simulink model "Linearized_system_simulink"  (R2023b)
settings: Solver=VariableStepAuto  StartTime=0.0  StopTime=100  RelTol=1e-3
values from neighbouring files (symbols this model uses):
  K = place(A,B,[-1, -2, -3, -4])    [Linearized_system.m]
  theta0 = 60000/(m*g)    (= 0.0784129224496)    [Linearized_system.m]
  v0 = 840/3.6    (= 233.333333333)    [Linearized_system.m]
  w0 = 0    [Linearized_system.m]
settings Model: Creator=nasir  LastModifiedBy=nasir

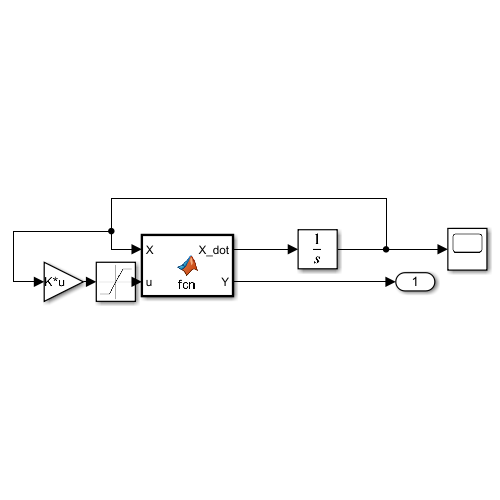
[thumbnail: Simulink's stored preview of the top-level diagram]
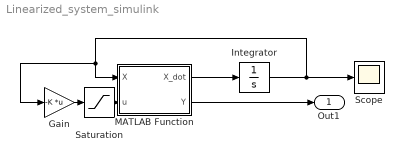
== system Linearized_system_simulink ==
  Gain : Gain  Gain=-K  Multiplication=Matrix(K*u)
  Integrator : Integrator  InitialCondition=[v0 w0 theta0 0.05]
  MATLAB Function : MATLAB Function  TreatAsAtomicUnit=on
  Saturation : Saturate  UpperLimit=[200000 900000 300000]  LowerLimit=[0 600000 -300000]
  Scope : Scope
  Out1 : Outport
  wires:
  MATLAB Function/2(Y) -> Out1/1
  Integrator/1 -> Gain/1, MATLAB Function/1(X), Scope/1
  MATLAB Function/1(X_dot) -> Integrator/1
  Gain/1 -> Saturation/1
  Saturation/1 -> MATLAB Function/2(u)

== matlab function Linearized_system_simulink/MATLAB Function ==
  data: X input; u input; X_dot output; Y output
function [X_dot, Y]= fcn(X, u)
%#codegen
m = 78000;
Iy = 9*10e6;
g = 9.81;

v0 = 840/3.6;
w0 = 0;
theta0 = 60000/(m*g);
q0 = 0;

A = [0 -q0 -g*cos(theta0) -w0;
    q0 0 g*sin(theta0) v0;
    0 0 0 1;
    0 0 0 0];

B = [1/m 0 0;
    0 1/m 0;
    0 0 0;
    0 0 1/Iy];

C = [0 0 1 0;
    0 0 0 1];

D = [0 0 0;
    0 0 0];

X_dot = A*X+B*u

Y = C*X + D*u
